simulink model "sys_main"  (R2014b)
settings: Solver=ode3  StartTime=0.0  StopTime=inf  FixedStep=1e-6  RelTol=1e-3
undefined symbols (not defined in the file or in its folder): serial
libraries: instrumentlib x2
settings Model: Creator=user3  LastModifiedBy=user3
settings SolverCC: AutoInsertRateTranBlk=on

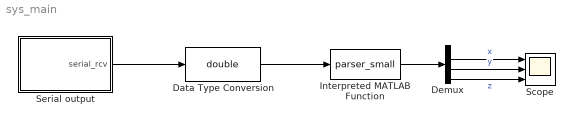
== system sys_main ==
  Data Type Conversion : DataTypeConversion  OutDataTypeStr=double
  Demux : Demux
  Interpreted MATLAB Function : MATLABFcn  MATLABFcn=parser_small
  Scope : Scope  NumInputPorts=3
      settings: ShowLegends=on  YMin=-10~-10~-10  YMax=10~10~10  MaxDataPoints=10000
  Serial output : Subsystem
  wires:
  Serial output/1(serial_rcv) -> Data Type Conversion/1
  Data Type Conversion/1 -> Interpreted MATLAB Function/1
  Interpreted MATLAB Function/1 -> Demux/1
  Demux/3 -> Scope/2  "y"
  Demux/2 -> Scope/1  "x"
  Demux/4 -> Scope/3  "z"

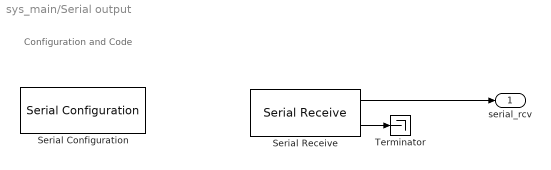
== system sys_main/Serial output ==
  note: Configuration and Code
  Serial Configuration : instrumentlib/Serial Configuration  Priority=-200000  ComPortMenu=COM6  ComPort=COM6  ObjConstructor=serial('COM6');  BaudRate=480900  DataBits=8  Parity=none  StopBits=1  FlowControl=none  Timeout=5  ByteOrder=LittleEndian
  Serial Receive : instrumentlib/Serial Receive  ComPortMenu=COM6  ComPort=COM6  ObjConstructor=serial('COM6');  Header=#:_  Terminator=<none>  DataSize="[772    1]"  DataType=uint8  EnableBlockingMode=off  ActionDataUnavailable=Output last received value  CustomValue=0  SampleTime=50e-3
  Terminator : Terminator
  serial_rcv : Outport
  wires:
  Serial Receive/2 -> Terminator/1
  Serial Receive/1 -> serial_rcv/1
